simulink model "ex6p3-closedLoop"  (R2016b)
settings: Solver=VariableStepAuto  StartTime=0.0  StopTime=9  RelTol=1e-3
libraries: powerlib x12, simulink x7, powerlib_meascontrol x1
settings Model: Creator=user  LastModifiedBy=user

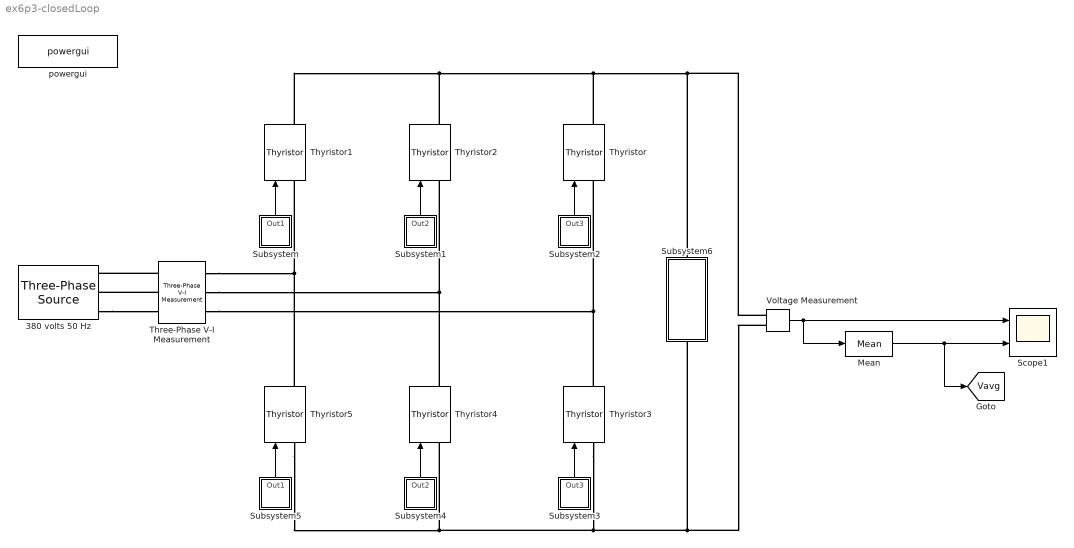
== system ex6p3-closedLoop ==
  380 volts 50 Hz : powerlib/Electrical Sources/Three-Phase Source  InternalConnection=Yg  VoltagePhases=off  Voltage=380  PhaseAngle=0  Voltage_phases=[25e3 25e3 25e3]/sqrt(3)  PhaseAngles_phases=[0 -120 +120]  Frequency=50  NonIdealSource=off  SpecifyImpedance=off  Resistance=0.8929  Inductance=16.58e-3  ShortCircuitLevel=100e6  BaseVoltage=25e3  XRratio=7  BusType=swing  Pref=10e3  Qref=0  Prefabc=[10e3, 10e3, 10e3]  Qrefabc=[0, 0, 0]  Qmin=-inf  Qmax=inf
  Mean : powerlib_meascontrol/Measurements/Mean  Freq=60  Vinit=0  Ts=0
  Scope1 : Scope  NumInputPorts=2
  Subsystem : Subsystem
  Subsystem1 : Subsystem
  Subsystem2 : Subsystem
  Subsystem3 : Subsystem
  Subsystem4 : Subsystem
  Subsystem5 : Subsystem
  Subsystem6 : Subsystem
  Three-Phase V-I Measurement : powerlib/Measurements/Three-Phase V-I Measurement  VoltageMeasurement=phase-to-ground  SetLabelV=on  LabelV=Vabc  Vpu=off  VpuLL=off  CurrentMeasurement=yes  SetLabelI=on  LabelI=Iabc  Ipu=off  Pbase=100e6  Vbase=500e3  OutputType=Complex  PhasorSimulation=off  PSBequivalent=0
  Thyristor{,1..5} (6 alike) : powerlib/Power Electronics/Thyristor  Ron=0.001  Lon=0  Vf=0.8  IC=0  Rs=500  Cs=250e-9  Measurements=on
  Voltage Measurement : powerlib/Measurements/Voltage Measurement  PhasorSimulation=off  OutputType=Complex  PSBequivalent=0
  powergui : powerlib/powergui  Priority=1  SimulationMode=Discrete  SolverType=Tustin/Backward Euler (TBE)  SampleTime=5e-5  frequency=60  SPID=off  DisableSnubberDevices=off  DisableRonSwitches=off  DisableVfSwitches=off  SwTol=0  DisplayEquations=off  Interpol=off  ExternalGateDelay=off  methode=off  Ts=10  FunctionMessages=off  echomessages=off  HookPort=off  EnableUseOfTLC=off  x0status=blocks  frequencyindice=0  Pbase=100e6  ErrMax=1e-4  Iterations=50  UnitsV=kV  UnitsW=MW  buscounter=0  RestoreLinks=warning  ResistiveCurrentMeasurement=off  Frange=[0:2:500]  Ylog=off  Xlog=on  ShowGrid=off  save=off  variable=ZData  structure=ScopeData  ZoomFFT=off  StartTime=0.08  cycles=2  DisplayStyle=1  fundamental=50  FreqAxis=off  MaxFrequency=1000  frequencyindicesteady=1  RmsSteady=1  display=off
  tag scope: Vavg=global
  wires:
  Voltage Measurement/1 -> Scope1/1, Mean/1
  Mean/1 -> [Vavg], Scope1/2
  Subsystem/1(Out1) -> Thyristor1/1
  Subsystem2/1(Out3) -> Thyristor/1
  Subsystem1/1(Out2) -> Thyristor2/1
  Subsystem3/1(Out3) -> Thyristor3/1
  Subsystem4/1(Out2) -> Thyristor4/1
  Subsystem5/1(Out1) -> Thyristor5/1
  connections:
  Thyristor2/LConn1 -- Thyristor4/RConn1 -- Three-Phase V-I Measurement/RConn2
  Thyristor/LConn1 -- Thyristor3/RConn1 -- Three-Phase V-I Measurement/RConn3
  Thyristor1/LConn1 -- Thyristor5/RConn1 -- Three-Phase V-I Measurement/RConn1
  Subsystem6/RConn1 -- Voltage Measurement/LConn2 -- Thyristor3/LConn1 -- Thyristor5/LConn1 -- Thyristor4/LConn1
  Voltage Measurement/LConn1 -- Subsystem6/LConn1 -- Thyristor/RConn1 -- Thyristor2/RConn1 -- Thyristor1/RConn1
  380 volts 50 Hz/RConn3 -- Three-Phase V-I Measurement/LConn3
  Three-Phase V-I Measurement/LConn2 -- 380 volts 50 Hz/RConn2
  Three-Phase V-I Measurement/LConn1 -- 380 volts 50 Hz/RConn1

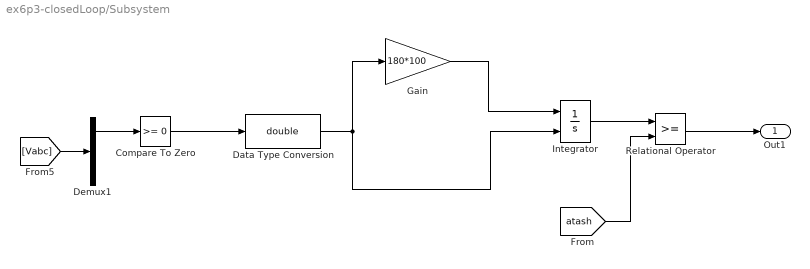
== system ex6p3-closedLoop/Subsystem ==
  Compare To Zero : simulink/Logic and Bit Operations/Compare To Zero  relop=>=  OutDataTypeStr=boolean
  Data Type Conversion : DataTypeConversion  OutDataTypeStr=double
  Demux1 : Demux  Outputs=3
  Gain : Gain  Gain=180*100
  Integrator : Integrator  ExternalReset=falling
  Relational Operator : RelationalOperator  OutDataTypeStr=boolean  RndMeth=Simplest
  Out1 : Outport
  wires:
  [Vabc] -> Demux1/1
  Gain/1 -> Integrator/1
  Integrator/1 -> Relational Operator/1
  Relational Operator/1 -> Out1/1
  Data Type Conversion/1 -> Gain/1, Integrator/2
  Compare To Zero/1 -> Data Type Conversion/1
  Demux1/1 -> Compare To Zero/1
  [atash] -> Relational Operator/2

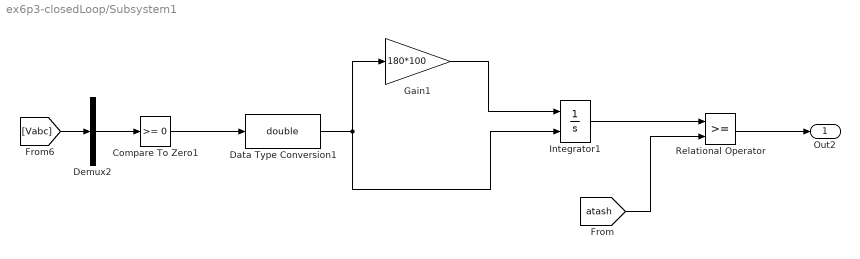
== system ex6p3-closedLoop/Subsystem1 ==
  Compare To Zero1 : simulink/Logic and Bit Operations/Compare To Zero  relop=>=  OutDataTypeStr=boolean
  Data Type Conversion1 : DataTypeConversion  OutDataTypeStr=double
  Demux2 : Demux  Outputs=3
  Gain1 : Gain  Gain=180*100
  Integrator1 : Integrator  ExternalReset=falling
  Relational Operator : RelationalOperator  OutDataTypeStr=boolean  RndMeth=Simplest
  Out2 : Outport
  wires:
  Demux2/2 -> Compare To Zero1/1
  Data Type Conversion1/1 -> Gain1/1, Integrator1/2
  Compare To Zero1/1 -> Data Type Conversion1/1
  Gain1/1 -> Integrator1/1
  [Vabc] -> Demux2/1
  Integrator1/1 -> Relational Operator/1
  Relational Operator/1 -> Out2/1
  [atash] -> Relational Operator/2

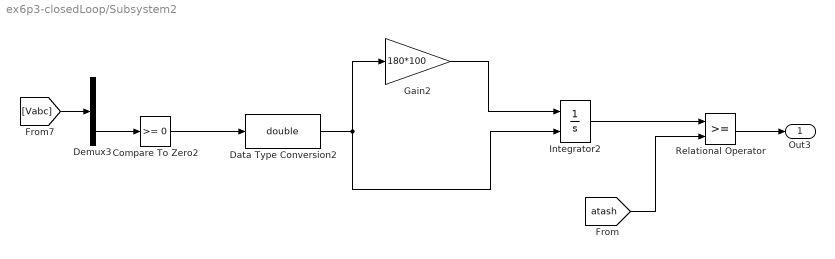
== system ex6p3-closedLoop/Subsystem2 ==
  Compare To Zero2 : simulink/Logic and Bit Operations/Compare To Zero  relop=>=  OutDataTypeStr=boolean
  Data Type Conversion2 : DataTypeConversion  OutDataTypeStr=double
  Demux3 : Demux  Outputs=3
  Gain2 : Gain  Gain=180*100
  Integrator2 : Integrator  ExternalReset=falling
  Relational Operator : RelationalOperator  OutDataTypeStr=boolean  RndMeth=Simplest
  Out3 : Outport
  wires:
  Data Type Conversion2/1 -> Gain2/1, Integrator2/2
  Compare To Zero2/1 -> Data Type Conversion2/1
  Gain2/1 -> Integrator2/1
  [Vabc] -> Demux3/1
  Demux3/3 -> Compare To Zero2/1
  Integrator2/1 -> Relational Operator/1
  Relational Operator/1 -> Out3/1
  [atash] -> Relational Operator/2

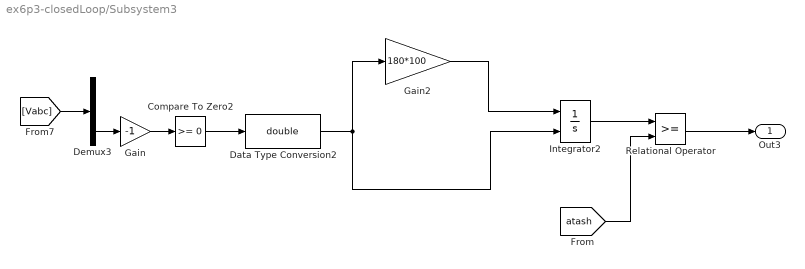
== system ex6p3-closedLoop/Subsystem3 ==
  Compare To Zero2 : simulink/Logic and Bit Operations/Compare To Zero  relop=>=  OutDataTypeStr=boolean
  Data Type Conversion2 : DataTypeConversion  OutDataTypeStr=double
  Demux3 : Demux  Outputs=3
  Gain : Gain  Gain=-1
  Gain2 : Gain  Gain=180*100
  Integrator2 : Integrator  ExternalReset=falling
  Relational Operator : RelationalOperator  OutDataTypeStr=boolean  RndMeth=Simplest
  Out3 : Outport
  wires:
  Data Type Conversion2/1 -> Gain2/1, Integrator2/2
  Compare To Zero2/1 -> Data Type Conversion2/1
  Gain2/1 -> Integrator2/1
  [Vabc] -> Demux3/1
  Demux3/3 -> Gain/1
  Gain/1 -> Compare To Zero2/1
  Integrator2/1 -> Relational Operator/1
  Relational Operator/1 -> Out3/1
  [atash] -> Relational Operator/2

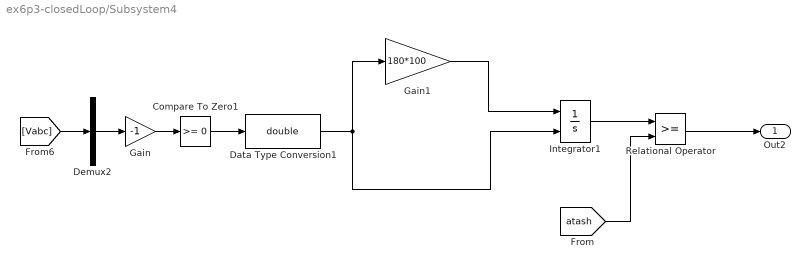
== system ex6p3-closedLoop/Subsystem4 ==
  Compare To Zero1 : simulink/Logic and Bit Operations/Compare To Zero  relop=>=  OutDataTypeStr=boolean
  Data Type Conversion1 : DataTypeConversion  OutDataTypeStr=double
  Demux2 : Demux  Outputs=3
  Gain : Gain  Gain=-1
  Gain1 : Gain  Gain=180*100
  Integrator1 : Integrator  ExternalReset=falling
  Relational Operator : RelationalOperator  OutDataTypeStr=boolean  RndMeth=Simplest
  Out2 : Outport
  wires:
  Data Type Conversion1/1 -> Gain1/1, Integrator1/2
  Compare To Zero1/1 -> Data Type Conversion1/1
  Gain1/1 -> Integrator1/1
  [Vabc] -> Demux2/1
  Demux2/2 -> Gain/1
  Gain/1 -> Compare To Zero1/1
  Integrator1/1 -> Relational Operator/1
  Relational Operator/1 -> Out2/1
  [atash] -> Relational Operator/2

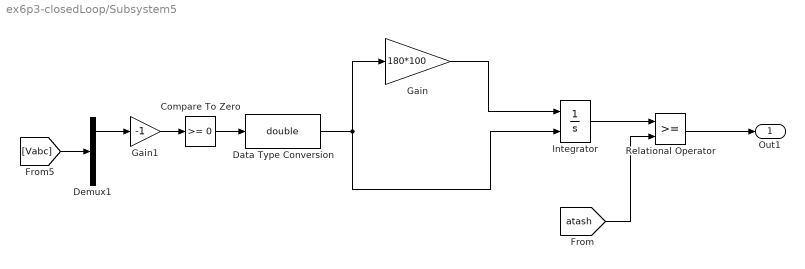
== system ex6p3-closedLoop/Subsystem5 ==
  Compare To Zero : simulink/Logic and Bit Operations/Compare To Zero  relop=>=  OutDataTypeStr=boolean
  Data Type Conversion : DataTypeConversion  OutDataTypeStr=double
  Demux1 : Demux  Outputs=3
  Gain : Gain  Gain=180*100
  Gain1 : Gain  Gain=-1
  Integrator : Integrator  ExternalReset=falling
  Relational Operator : RelationalOperator  OutDataTypeStr=boolean  RndMeth=Simplest
  Out1 : Outport
  wires:
  [Vabc] -> Demux1/1
  Gain/1 -> Integrator/1
  Data Type Conversion/1 -> Gain/1, Integrator/2
  Compare To Zero/1 -> Data Type Conversion/1
  Demux1/1 -> Gain1/1
  Gain1/1 -> Compare To Zero/1
  Integrator/1 -> Relational Operator/1
  Relational Operator/1 -> Out1/1
  [atash] -> Relational Operator/2

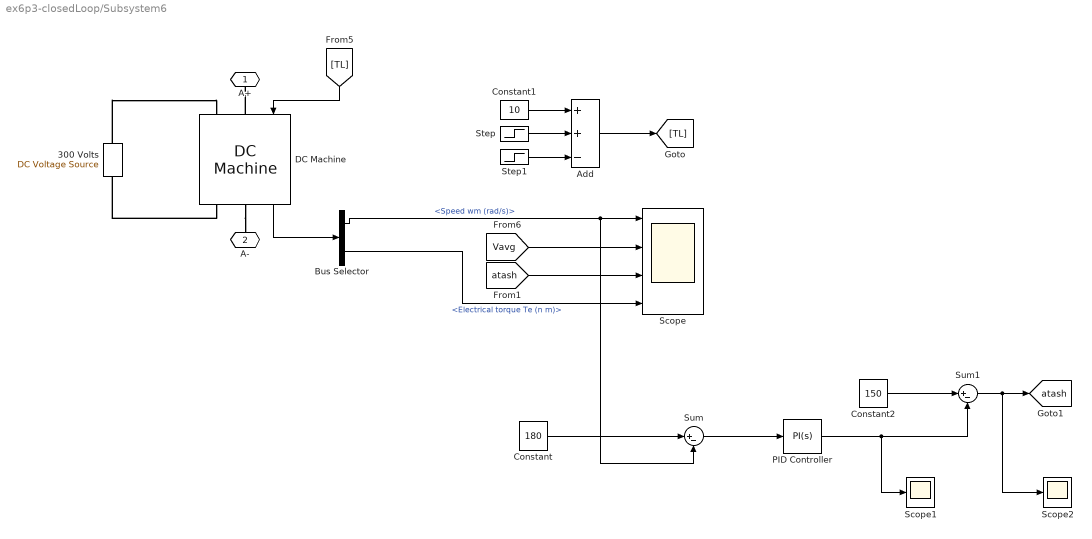
== system ex6p3-closedLoop/Subsystem6 ==
  300 Volts : powerlib/Electrical Sources/DC Voltage Source  Amplitude=300  Measurements=None
  Add : Sum  Inputs=++-
  Bus Selector : BusSelector  OutputSignals=Speed wm (rad/s),Electrical torque Te (n m)
  Constant : Constant  Value=180
  Constant1 : Constant  Value=10
  Constant2 : Constant  Value=150
  DC Machine : powerlib/Machines/DC Machine  PresetModel=03: 5HP 500V 1750RPM Field:300V  MechanicalLoad=Torque TL  FieldType=Wound  ShowDetailedParameters=on  MeasurementBus=off  RLa=[11.2 0.1215]  RLf=[281.3 156]  Laf=1.976  MachineConstant=Torque constant (N.m/A)  Ke=1.8  Kt=1.8  J=0.02215  Bm=0.002953  Tf=0.5161  w0=1  Ifinit=1  TsPowergui=0  TsBlock=-1
  PID Controller : simulink/Continuous/PID Controller  Controller=PI  TimeDomain=Continuous-time  SampleTime=-1  IntegratorMethod=Forward Euler  FilterMethod=Forward Euler  Form=Parallel  UseFilter=on  ControllerParametersSource=internal  P=3  I=20  D=0  N=100  InitialConditionSource=internal  InitialConditionForIntegrator=0  InitialConditionForFilter=0  ExternalReset=none  LimitOutput=off  UpperSaturationLimit=inf  LowerSaturationLimit=-inf  LinearizeAsGain=on  AntiWindupMode=none  Kb=1  TrackingMode=off  Kt=1  PParamMin=[]  PParamMax=[]  IParamMin=[]  IParamMax=[]  DParamMin=[]  DParamMax=[]  NParamMin=[]  NParamMax=[]  KbParamMin=[]  KbParamMax=[]  KtParamMin=[]  KtParamMax=[]  POutMin=[]  POutMax=[]  IOutMin=[]  IOutMax=[]  DOutMin=[]  DOutMax=[]  NOutMin=[]  NOutMax=[]  KbOutMin=[]  KbOutMax=[]  KtOutMin=[]  KtOutMax=[]  IntegratorOutMin=[]  IntegratorOutMax=[]  FilterOutMin=[]  FilterOutMax=[]  SumOutMin=[]  SumOutMax=[]  SumI1OutMin=[]  SumI1OutMax=[]  SumI2OutMin=[]  SumI2OutMax=[]  SumI3OutMin=[]  SumI3OutMax=[]  SumDOutMin=[]  SumDOutMax=[]  SaturationOutMin=[]  SaturationOutMax=[]  IntegratorContinuousStateAttributes=''  IntegratorStateMustResolveToSignalObject=off  IntegratorRTWStateStorageClass=Auto  FilterContinuousStateAttributes=''  FilterStateMustResolveToSignalObject=off  FilterRTWStateStorageClass=Auto  DifferentiatorICPrevScaledInput=0  DifferentiatorOutMin=[]  DifferentiatorOutMax=[]
  Scope : Scope  NumInputPorts=4
  Scope1 : Scope
  Scope2 : Scope
  Step : Step  Time=3  After=5  SampleTime=0
  Step1 : Step  Time=6  After=10  SampleTime=0
  Sum : Sum  Inputs=|+-
  Sum1 : Sum  Inputs=|+-
  A+ : PMIOPort  Port=1  Side=Left
  A- : PMIOPort  Port=2  Side=Right
  tag scope: atash=global
  wires:
  DC Machine/1 -> Bus Selector/1
  Step1/1 -> Add/3
  Bus Selector/1 -> Sum/2, Scope/1  "<Speed wm (rad/s)>"
  [Vavg] -> Scope/2
  Step/1 -> Add/2
  Add/1 -> [TL]
  Constant1/1 -> Add/1
  [TL] -> DC Machine/1
  [atash] -> Scope/3
  Bus Selector/2 -> Scope/4  "<Electrical torque Te (n m)>"
  Constant/1 -> Sum/1
  Sum/1 -> PID Controller/1
  PID Controller/1 -> Scope1/1, Sum1/2
  Constant2/1 -> Sum1/1
  Sum1/1 -> Scope2/1, [atash]
  connections:
  DC Machine/LConn1 -- A+/RConn1
  DC Machine/RConn1 -- A-/RConn1
  DC Machine/RConn2 -- 300 Volts/LConn1
  300 Volts/RConn1 -- DC Machine/LConn2
